simulink model "svm_tracking_1pred"  (Simulink 8.6)
settings: Solver=VariableStepAuto  StartTime=0.0  StopTime=10.0  RelTol=1e-3
values from neighbouring files (symbols this model uses):
  M_psderivative = ss(blkdiag(T_psderivative, T_psderivative, T_psderivative))    [svm_buildLinearControllers.m]
  My = ss(tf([eye(6) -eye(6)]))    [svm_buildLinearControllers.m]
  Mz = ss(tf([pickP, -pickP]))    [svm_buildLinearControllers.m]
  turbulence2loadfactors = blkdiag(T_w2nx, T_w2nz)    [svm_buildLinearControllers.m]
settings Model: Creator=j.bolting  LastModifiedBy=j.bolting
settings DataIOCC: SaveFormat=StructureWithTime  SignalLoggingSaveFormat=Dataset
settings OptimizationCC: BlockReduction=off  DefaultParameterBehavior=Inlined  BufferReuse=off  ExpressionDepthLimit=128
settings DebuggingCC: AlgebraicLoopMsg=none  UnderspecifiedInitializationDetection=Simplified  MergeDetectMultiDrivingBlocksExec=error  SolverPrmCheckMsg=none  FcnCallInpInsideContextMsg=EnableAllAsError  UnconnectedInputMsg=none  UnconnectedOutputMsg=none  UnconnectedLineMsg=none  StateNameClashWarn=none  InitInArrayFormatMsg=none
settings HardwareCC: ProdBitPerPointer=64  ProdLargestAtomicFloat=Float  ProdIntDivRoundTo=Zero  ProdEndianess=LittleEndian  ProdWordSize=64  ProdHWDeviceType=Intel->x86-64 (Windows64)
settings GRTTargetCC: GeneratePreprocessorConditionals=Use local settings  CombineOutputUpdateFcns=on  GRTInterface=off
settings ConfigComp: CovModelRefEnable=off

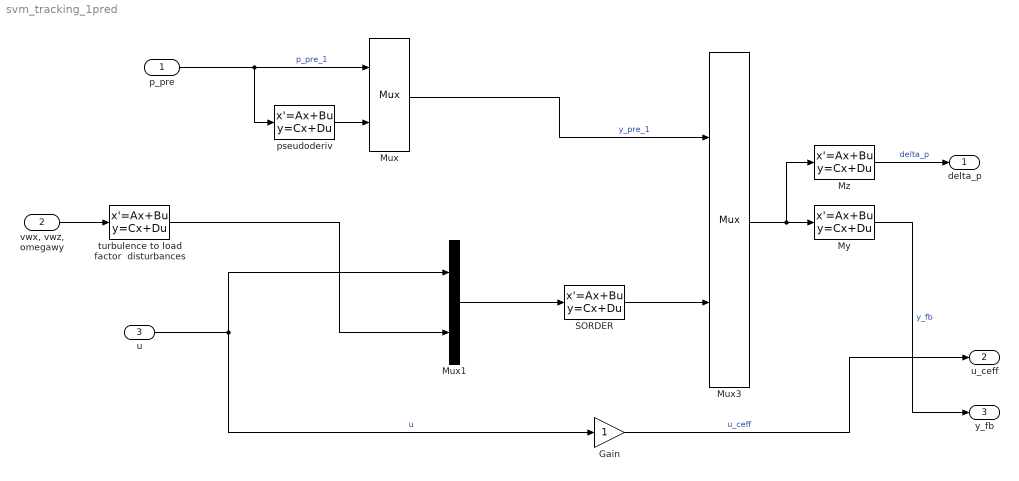
== system svm_tracking_1pred ==
  p_pre : Inport  PortDimensions=2
  "vwx, vwz, omegawy" : Inport  Port=2  PortDimensions=3
  u : Inport  Port=3  PortDimensions=2
  Gain : Gain
  Mux : Mux  Inputs=2
  Mux1 : Mux  Inputs=2
  Mux3 : Mux  Inputs=2
  My : StateSpace  A=My.a  B=My.b  C=My.c  D=My.d  X0=0
  Mz : StateSpace  A=Mz.a  B=Mz.b  C=Mz.c  D=Mz.d  X0=0
  SORDER : StateSpace  A=uavsim.svm.linearmodels.sorder_longi.airspeed_15.a  B=uavsim.svm.linearmodels.sorder_longi.airspeed_15.b  C=uavsim.svm.linearmodels.sorder_longi.airspeed_15.c  D=uavsim.svm.linearmodels.sorder_longi.airspeed_15.d  X0=0
  pseudoderiv : StateSpace  A=M_psderivative.a  B=M_psderivative.b  C=M_psderivative.c  D=M_psderivative.d  X0=0
  turbulence to load factor  disturbances : StateSpace  A=turbulence2loadfactors.a  B=turbulence2loadfactors.b  C=turbulence2loadfactors.c  D=turbulence2loadfactors.d  X0=0
  delta_p : Outport
  u_ceff : Outport  Port=2
  y_fb : Outport  Port=3
  wires:
  pseudoderiv/1 -> Mux/2
  p_pre/1 -> pseudoderiv/1, Mux/1  "p_pre_1"
  Mux/1 -> Mux3/1  "y_pre_1"
  SORDER/1 -> Mux3/2
  Mux3/1 -> Mz/1, My/1
  Mz/1 -> delta_p/1  "delta_p"
  My/1 -> y_fb/1  "y_fb"
  u/1 -> Gain/1, Mux1/1  "u"
  Mux1/1 -> SORDER/1
  Gain/1 -> u_ceff/1  "u_ceff"
  turbulence to load factor  disturbances/1 -> Mux1/2
  "vwx, vwz, omegawy"/1 -> turbulence to load factor  disturbances/1
